simulink model "simulationModel"  (Simulink 7.4)
settings: Solver=ode45  StartTime=0.0  StopTime=30  RelTol=1e-3
values from neighbouring files (symbols this model uses):
  qr = [xr', yr', thetar']    [computeReferenceFromLissajous.m]
  ur = [vr', dthetar']    [computeReferenceFromLissajous.m]
undefined symbols (not defined in the file or in its folder): b, l, M, n, N, omegaMax, p, Qbar, r, Rbar, S, T, theta0, thetaStd, x0, xStd, y0, yStd
libraries: aerolibutil x1
settings Model: Creator=MarcosRicardo  LastModifiedBy=MarcosRicardo

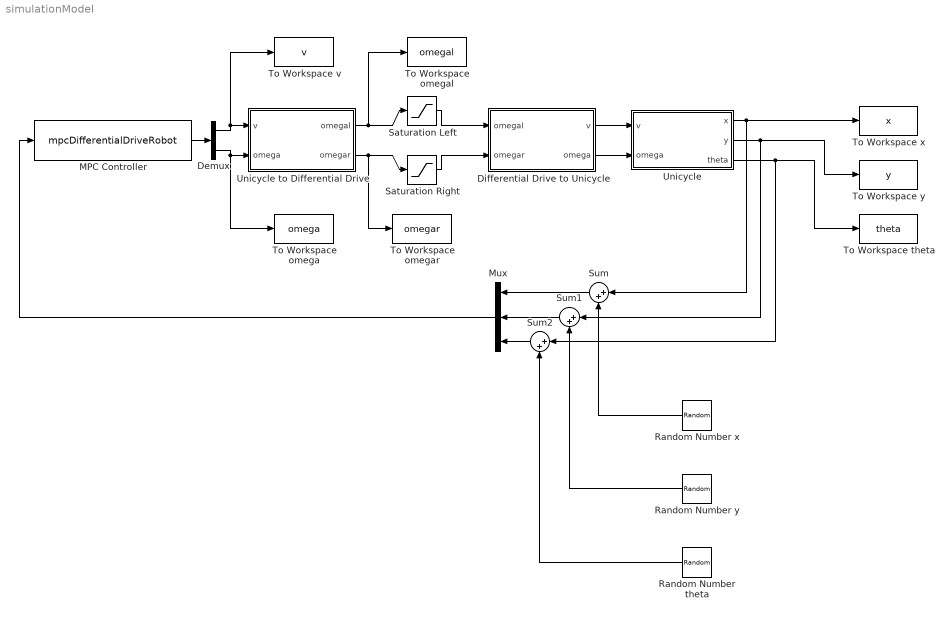
== system simulationModel ==
  Demux : Demux  Outputs=2
  Differential Drive to Unicycle : Subsystem
  MPC Controller : S-Function  FunctionName=mpcDifferentialDriveRobot  Parameters=qr,ur,Qbar,Rbar,S,b,p,n,M,N,T  EnableBusSupport=off
  Mux : Mux  Inputs=3
  Random Number theta : RandomNumber  Variance=thetaStd^2  Seed=3  SampleTime=T
  Random Number x : RandomNumber  Variance=xStd^2  Seed=1  SampleTime=T
  Random Number y : RandomNumber  Variance=yStd^2  Seed=2  SampleTime=T
  Saturation Left : Saturate  UpperLimit=omegaMax  LowerLimit=-omegaMax  OutDataType=fixdt(1, 16)  OutScaling=2^0
  Saturation Right : Saturate  UpperLimit=omegaMax  LowerLimit=-omegaMax  OutDataType=fixdt(1, 16)  OutScaling=2^0
  Sum : Sum  Inputs=|++  OutDataType=fixdt(1, 16)  OutScaling=2^0
  Sum1 : Sum  Inputs=|++  OutDataType=fixdt(1, 16)  OutScaling=2^0
  Sum2 : Sum  Inputs=|++  OutDataType=fixdt(1, 16)  OutScaling=2^0
  To Workspace omega : ToWorkspace  VariableName=omega  SampleTime=-1  SaveFormat=Structure With Time
  To Workspace omegal : ToWorkspace  VariableName=omegal  SampleTime=-1  SaveFormat=Structure With Time
  To Workspace omegar : ToWorkspace  VariableName=omegar  SampleTime=-1  SaveFormat=Structure With Time
  To Workspace theta : ToWorkspace  VariableName=theta  SampleTime=-1  SaveFormat=Structure With Time
  To Workspace v : ToWorkspace  VariableName=v  SampleTime=-1  SaveFormat=Structure With Time
  To Workspace x : ToWorkspace  VariableName=x  SampleTime=-1  SaveFormat=Structure With Time
  To Workspace y : ToWorkspace  VariableName=y  SampleTime=-1  SaveFormat=Structure With Time
  Unicycle : Subsystem
  Unicycle to Differential Drive : Subsystem
  wires:
  Unicycle/1(x) -> To Workspace x/1, Sum/1
  Unicycle/2(y) -> To Workspace y/1, Sum1/1
  Unicycle/3(theta) -> To Workspace theta/1, Sum2/1
  Unicycle to Differential Drive/1(omegal) -> Saturation Left/1, To Workspace omegal/1
  Unicycle to Differential Drive/2(omegar) -> Saturation Right/1, To Workspace omegar/1
  Mux/1 -> MPC Controller/1
  Saturation Left/1 -> Differential Drive to Unicycle/1(omegal)
  Saturation Right/1 -> Differential Drive to Unicycle/2(omegar)
  MPC Controller/1 -> Demux/1
  Demux/1 -> Unicycle to Differential Drive/1(v), To Workspace v/1
  Demux/2 -> Unicycle to Differential Drive/2(omega), To Workspace omega/1
  Differential Drive to Unicycle/1(v) -> Unicycle/1(v)
  Differential Drive to Unicycle/2(omega) -> Unicycle/2(omega)
  Sum/1 -> Mux/1
  Random Number x/1 -> Sum/2
  Sum1/1 -> Mux/2
  Random Number y/1 -> Sum1/2
  Sum2/1 -> Mux/3
  Random Number theta/1 -> Sum2/2

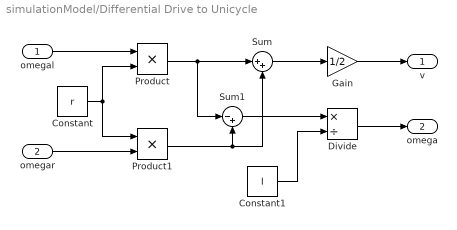
== system simulationModel/Differential Drive to Unicycle ==
  omegal : Inport  OutDataType=fixdt(1, 16)  OutScaling=2^0
  omegar : Inport  Port=2  OutDataType=fixdt(1, 16)  OutScaling=2^0
  Constant : Constant  Value=r  OutDataType=fixdt(1, 16)  OutScaling=2^0
  Constant1 : Constant  Value=l  OutDataType=fixdt(1, 16)  OutScaling=2^0
  Divide : Product  Inputs=*/  OutDataType=fixdt(1, 16)  OutScaling=2^-10
  Gain : Gain  Gain=1/2  ParameterDataType=fixdt(1, 16)  ParameterScaling=2^0  OutDataType=fixdt(1, 16)  OutScaling=2^0
  Product : Product  OutDataType=fixdt(1, 16)  OutScaling=2^0  RndMeth=Zero
  Product1 : Product  OutDataType=fixdt(1, 16)  OutScaling=2^0  RndMeth=Zero
  Sum : Sum  Inputs=|++  OutDataType=fixdt(1, 16)  OutScaling=2^0
  Sum1 : Sum  Inputs=|-+  OutDataType=fixdt(1, 16)  OutScaling=2^0
  v : Outport  OutDataType=fixdt(1, 16)  OutScaling=2^0
  omega : Outport  Port=2  OutDataType=fixdt(1, 16)  OutScaling=2^0
  wires:
  Constant/1 -> Product/2, Product1/1
  omegal/1 -> Product/1
  omegar/1 -> Product1/2
  Product/1 -> Sum/1, Sum1/1
  Product1/1 -> Sum/2, Sum1/2
  Sum/1 -> Gain/1
  Sum1/1 -> Divide/1
  Constant1/1 -> Divide/2
  Divide/1 -> omega/1
  Gain/1 -> v/1

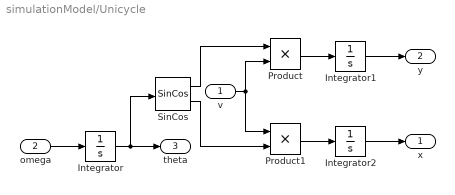
== system simulationModel/Unicycle ==
  v : Inport  OutDataType=fixdt(1, 16)  OutScaling=2^0
  omega : Inport  Port=2  OutDataType=fixdt(1, 16)  OutScaling=2^0
  Integrator : Integrator  InitialCondition=theta0
  Integrator1 : Integrator  InitialCondition=y0
  Integrator2 : Integrator  InitialCondition=x0
  Product : Product  OutDataType=fixdt(1, 16)  OutScaling=2^0  RndMeth=Zero
  Product1 : Product  OutDataType=fixdt(1, 16)  OutScaling=2^0  RndMeth=Zero
  SinCos : aerolibutil/SinCos  SystemSampleTime=-1
  x : Outport  OutDataType=fixdt(1, 16)  OutScaling=2^0
  y : Outport  Port=2  OutDataType=fixdt(1, 16)  OutScaling=2^0
  theta : Outport  Port=3  OutDataType=fixdt(1, 16)  OutScaling=2^0
  wires:
  omega/1 -> Integrator/1
  Integrator/1 -> SinCos/1, theta/1
  v/1 -> Product/2, Product1/1
  SinCos/1 -> Product/1
  SinCos/2 -> Product1/2
  Product/1 -> Integrator1/1
  Integrator1/1 -> y/1
  Product1/1 -> Integrator2/1
  Integrator2/1 -> x/1

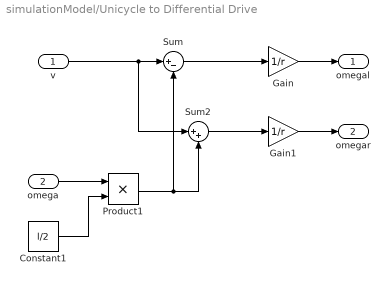
== system simulationModel/Unicycle to Differential Drive ==
  v : Inport  OutDataType=fixdt(1, 16)  OutScaling=2^0
  omega : Inport  Port=2  OutDataType=fixdt(1, 16)  OutScaling=2^0
  Constant1 : Constant  Value=l/2  OutDataType=fixdt(1, 16)  OutScaling=2^0
  Gain : Gain  Gain=1/r  ParameterDataType=fixdt(1, 16)  ParameterScaling=2^0  OutDataType=fixdt(1, 16)  OutScaling=2^0
  Gain1 : Gain  Gain=1/r  ParameterDataType=fixdt(1, 16)  ParameterScaling=2^0  OutDataType=fixdt(1, 16)  OutScaling=2^0
  Product1 : Product  OutDataType=fixdt(1, 16)  OutScaling=2^0  RndMeth=Zero
  Sum : Sum  Inputs=|+-  OutDataType=fixdt(1, 16)  OutScaling=2^0
  Sum2 : Sum  Inputs=|++  OutDataType=fixdt(1, 16)  OutScaling=2^0
  omegal : Outport  OutDataType=fixdt(1, 16)  OutScaling=2^0
  omegar : Outport  Port=2  OutDataType=fixdt(1, 16)  OutScaling=2^0
  wires:
  v/1 -> Sum/1, Sum2/1
  omega/1 -> Product1/1
  Constant1/1 -> Product1/2
  Product1/1 -> Sum/2, Sum2/2
  Sum/1 -> Gain/1
  Sum2/1 -> Gain1/1
  Gain1/1 -> omegar/1
  Gain/1 -> omegal/1
